simulink model "deadReckoningSF_soln"  (R2017a)
settings: Solver=VariableStepAuto  StartTime=0.0  StopTime=2000  RelTol=1e-3
PreLoadFcn:
  | robotParameters;
  | ticksPerRot = 360;
values from neighbouring files (symbols this model uses):
  wheelR = 0.052    [robotParameters.m]
libraries: simulink x2
settings Model: Creator=sseshadr  LastModifiedBy=shiremat

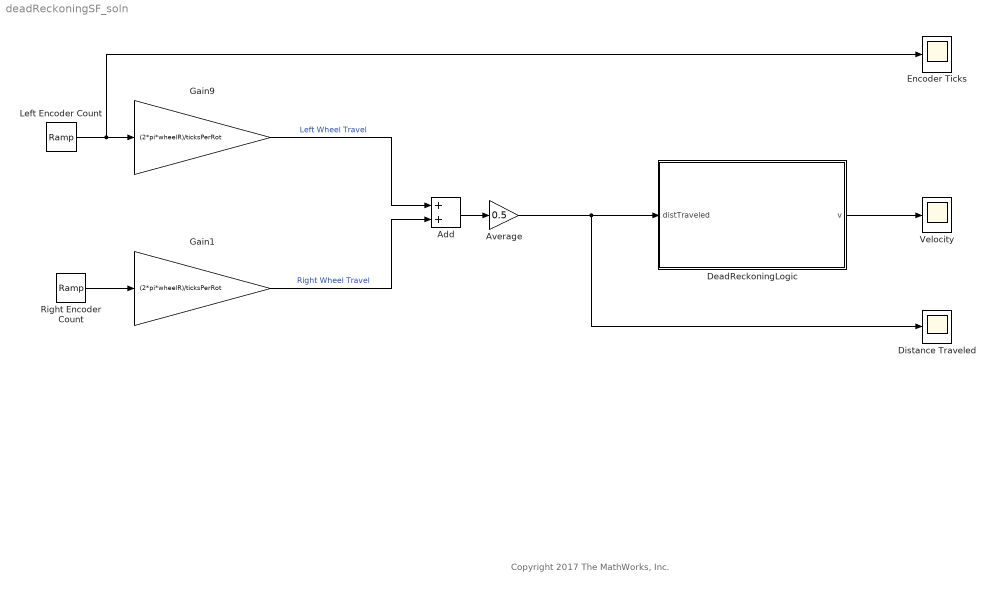
== system deadReckoningSF_soln ==
  note: Copyright 2017 The MathWorks, Inc.
  Add : Sum
  Average : Gain  Gain=0.5
  DeadReckoningLogic : Stateflow chart  TreatAsAtomicUnit=on
  Distance Traveled : Scope
  Encoder Ticks : Scope
  Gain1 : Gain  Gain=(2*pi*wheelR)/ticksPerRot
  Gain9 : Gain  Gain=(2*pi*wheelR)/ticksPerRot
  Left Encoder Count : simulink/Sources/Ramp  slope=1  start=0  X0=0
  Right Encoder Count : simulink/Sources/Ramp  slope=1  start=0  X0=0
  Velocity : Scope
  wires:
  Average/1 -> DeadReckoningLogic/1(distTraveled), Distance Traveled/1
  DeadReckoningLogic/1(v) -> Velocity/1
  Gain9/1 -> Add/1  "Left Wheel Travel"
  Right Encoder Count/1 -> Gain1/1
  Left Encoder Count/1 -> Gain9/1, Encoder Ticks/1
  Add/1 -> Average/1
  Gain1/1 -> Add/2  "Right Wheel Travel"

== stateflow chart deadReckoningSF_soln/DeadReckoningLogic ==
  state MoveForward
    entry:
    v = 0.1;
  state Stop
    entry:
    v = 0;
  (default) -> MoveForward : %Start Dead Reckoning
  MoveForward -> Stop : [distTraveled >= 1]
  data: v output; distTraveled input
